simulink model "mpsimulationv5_2"  (R2025a)
settings: Solver=ode45  StartTime=0.0  StopTime=50  MaxStep=0.1  RelTol=1e-3
undefined symbols (not defined in the file): gray
libraries: dspvision x1, slpidlib x1, autolibshared x1
settings Model: Creator=shipr  LastModifiedBy=bcb

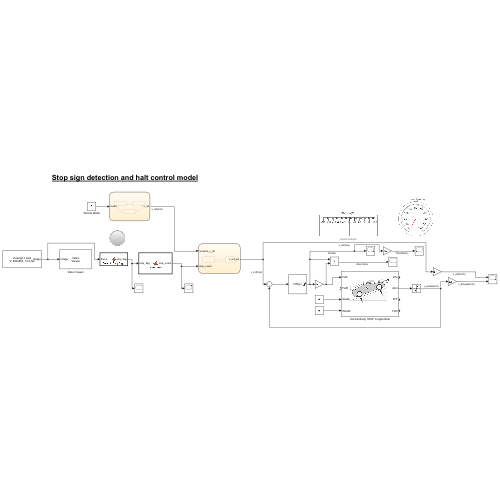
[thumbnail: Simulink's stored preview of the top-level diagram]
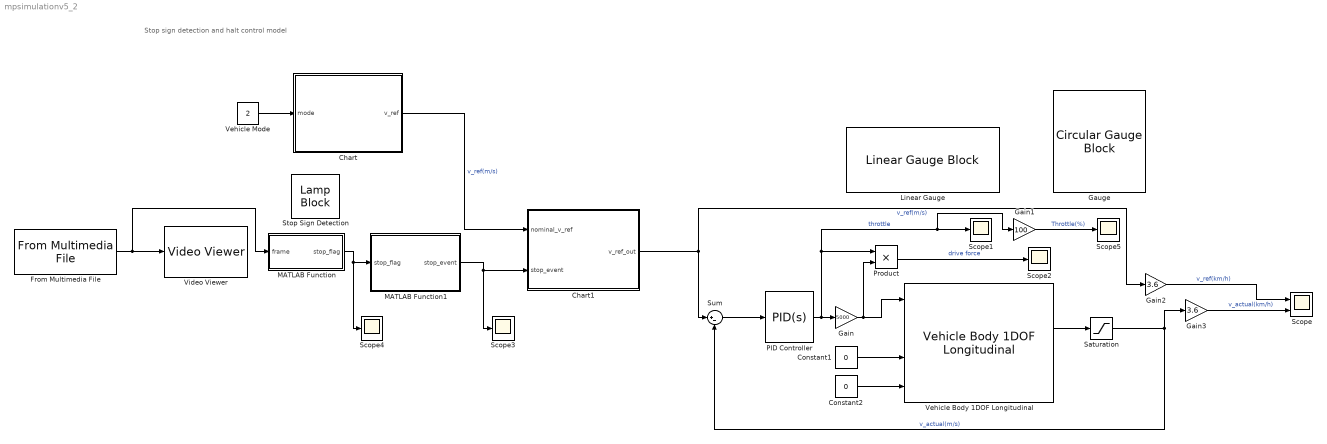
== system mpsimulationv5_2 ==
  note: Stop sign detection and halt control model
  Chart : Stateflow chart  TreatAsAtomicUnit=on
  Chart1 : Stateflow chart  TreatAsAtomicUnit=on
  Constant1 : Constant  Value=0
  Constant2 : Constant  Value=0
  From Multimedia File : dspvision/From Multimedia File  inputFilename=C:\Users\bcb\Downloads\stopsign1.mp4  readRange=[1 Inf]  loop=on  numPlays=inf  outputStreams=Video only  videoDataType=uint8  audioDataType=int16  inheritSampleTime=off  userDefinedSampleTime=0.1  noAudioOutput=off  isIntensityVideo=off  fourcc=RGB  colorVideoFormat=One multidimensional signal  outputEOF=off  dataOrg=Column-major  audioFrameSize=1024  computeAudioFrameSize=off  outSamplingMode=Sample based
      settings: LibrarySourceBlock=visionsources/From Multimedia File
  Gain : Gain  Gain=5000
  Gain1 : Gain  Gain=100
  Gain2 : Gain  Gain=3.6
  Gain3 : Gain  Gain=3.6
  Gauge : CircularGaugeBlock  FontColor=[0.0, 0.0, 0.0]
  Linear Gauge : LinearGaugeBlock  ScaleMin=-100  FontColor=[0.0, 0.0, 0.0]
  MATLAB Function : MATLAB Function  TreatAsAtomicUnit=on
  MATLAB Function1 : MATLAB Function  TreatAsAtomicUnit=on
  PID Controller : slpidlib/PID Controller  Controller=PID  Form=Parallel  TimeDomain=Continuous-time  UseExternalTs=off  SampleTime=-1  IntegratorMethod=Forward Euler  FilterMethod=Forward Euler  ControllerParametersSource=internal  P=1  I=0.1  UseKiTs=off  D=0  UseExternalDerivativeSource=off  N=100  UseFilter=on  TunerSelectOption=Transfer Function Based (PID Tuner App)  InitialConditionSource=internal  InitialConditionForIntegrator=0  InitialConditionForFilter=0  DifferentiatorICPrevScaledInput=0  ExternalReset=none  TrackingMode=off  Kt=1  LimitOutput=on  SatLimitsSource=internal  UpperSaturationLimit=1  LowerSaturationLimit=-1  LinearizeAsGain=on  AntiWindupMode=back-calculation  Kb=1  LimitIntegrator=off  UpperIntegratorSaturationLimit=inf  LowerIntegratorSaturationLimit=-inf  POutMin=[]  POutMax=[]  IOutMin=[]  IOutMax=[]  DOutMin=[]  DOutMax=[]  NOutMin=[]  NOutMax=[]  SumOutMin=[]  SumOutMax=[]  SaturationOutMin=[]  SaturationOutMax=[]  PParamMin=[]  PParamMax=[]  IParamMin=[]  IParamMax=[]  DParamMin=[]  DParamMax=[]  NParamMin=[]  NParamMax=[]  KbParamMin=[]  KbParamMax=[]  KtParamMin=[]  KtParamMax=[]  KbOutMin=[]  KbOutMax=[]  KtOutMin=[]  KtOutMax=[]  IntegratorOutMin=[]  IntegratorOutMax=[]  FilterOutMin=[]  FilterOutMax=[]  SumI1OutMin=[]  SumI1OutMax=[]  SumI2OutMin=[]  SumI2OutMax=[]  SumI3OutMin=[]  SumI3OutMax=[]  SumI4OutMin=[]  SumI4OutMax=[]  SumDOutMin=[]  SumDOutMax=[]  DifferentiatorOutMin=[]  DifferentiatorOutMax=[]  FilterDiffOutCoefMin=[]  FilterDiffOutCoefMax=[]  ReciprocalOutMin=[]  ReciprocalOutMax=[]  SumDenOutMin=[]  SumDenOutMax=[]  SumNumOutMin=[]  SumNumOutMax=[]  DivideOutMin=[]  DivideOutMax=[]  UdiffTsProdOutMin=[]  UdiffTsProdOutMax=[]  NTsProdOutMin=[]  NTsProdOutMax=[]  UintegralTsProdOutMin=[]  UintegralTsProdOutMax=[]  UngainTsProdOutMin=[]  UngainTsProdOutMax=[]  ClampingZeroOutDataTypeStr=Inherit: Inherit via back propagation  ClampingZeroOutMin=[]  ClampingZeroOutMax=[]  FilterDenConstantOutDataTypeStr=Inherit: Inherit via back propagation  FilterDenConstantOutMin=[]  FilterDenConstantOutMax=[]  PCopyOutDataTypeStr=Inherit: Inherit via back propagation  PCopyOutMin=[]  PCopyOutMax=[]  NCopyOutDataTypeStr=Inherit: Inherit via back propagation  NCopyOutMin=[]  NCopyOutMax=[]  IntegratorContinuousStateAttributes=''  IntegratorStateMustResolveToSignalObject=off  IntegratorRTWStateStorageClass=Auto  FilterContinuousStateAttributes=''  FilterStateMustResolveToSignalObject=off  FilterRTWStateStorageClass=Auto  ParallelPVariant=InternalParameters  IdealPVariant=Disabled  IVariant=InternalParameters  DVariant=InternalParameters  IntegratorVariant=Continuous  SatVariant=Enabled  AWVariant=BackCalculation  PCopyVariant=Disabled  TRVariant=Disabled  FdbkBlocksVariant=Forward  IdealPFdbkVariant=Disabled  SatFdbkVariant=Disabled  DerivativeFilterVariant=ContFilter  NVariant=InternalParameters  NCopyVariant=Disabled  FilterICVariant=InternalICsFilter  IntegratorICVariant=InternalICs  ExternalResetVariant=Disabled  TRSumVariant=Passthrough  SumFdbkVariant=Disabled  SumVariant=Sum_PID  TsampFilterVariant=InternalTs  TsampNgainVariant=Passthrough  TsampIntegralVariant=Disabled_SignalSpec  ExternalSaturationOutDataTypeStr=Inherit: Same as second input  DerivativeSourceVariant=ErrorSignal  PreIntVariant=InternalPreInt
  Product : Product
  Saturation : Saturate  UpperLimit=41.6667  LowerLimit=0
  Scope : Scope  NumInputPorts=2
      settings: Title=Velocity vs Time  ShowGrid=off  ActiveDisplayYMinimum=-327.61362751002292  ActiveDisplayYMaximum=94.622504183369685  YLabel=Velocity(km/h)
  Scope{1..5} (5 alike) : Scope
      Scope1 settings: ActiveDisplayYMinimum=-0.18455559045226133  ActiveDisplayYMaximum=1.1935694095477389
      Scope2 settings: Title=Drive Force  ActiveDisplayYMinimum=-1685.3571517954197  ActiveDisplayYMaximum=6690.2406021108291  YLabel=Drive Force  DataLoggingVariableName=ScopeData2
      Scope3 settings: ActiveDisplayYMinimum=-1.0419685990338166  ActiveDisplayYMaximum=1.0580314009661835  DataLoggingVariableName=ScopeData3
      Scope4 settings: ActiveDisplayYMinimum=-1  ActiveDisplayYMaximum=1  DataLoggingVariableName=ScopeData4
      Scope5 settings: ActiveDisplayYMinimum=-125  ActiveDisplayYMaximum=125  YLabel=Throttle (%)  DataLoggingVariableName=ScopeData5
  Stop Sign Detection : LampBlock  Tag=Stop Sign Detection  LabelPosition=Hide  DefaultColor=[192.0, 192.0, 192.0]
  Sum : Sum  Inputs=|+-
  Vehicle Body 1DOF Longitudinal : autolibshared/Vehicle Body 1DOF Longitudinal  VariantControl=SL  extFMode=off  extMMode=off  extTamb=off  wind3D=off  aMode=2  NF=2  NR=2  m=1500  a=1.4  b=1.8  h=.35  Cd=0  Cl=0  Cpm=0  Af=2.2  x_o=0  xdot_o=0  Pabs=101325  T=293  g=9.81
      settings: LibrarySourceBlock=vehdynlibeom/Vehicle Body 1DOF Longitudinal
  Vehicle Mode : Constant  Value=2
  Video Viewer : VideoViewer  colormapValue=gray(256)  FigPos=[485 762 467 342]
  wires:
  Vehicle Mode/1 -> Chart/1(mode)
  Saturation/1 -> Gain3/1, Sum/2  "v_actual(m/s)"
  Vehicle Body 1DOF Longitudinal/2 -> Saturation/1
  PID Controller/1 -> Gain1/1, Scope1/1, Product/1, Gain/1  "throttle"
  Gain/1 -> Product/2, Vehicle Body 1DOF Longitudinal/1
  Constant1/1 -> Vehicle Body 1DOF Longitudinal/3
  Constant2/1 -> Vehicle Body 1DOF Longitudinal/4
  Product/1 -> Scope2/1  "drive force"
  From Multimedia File/1 -> MATLAB Function/1(frame), Video Viewer/1
  MATLAB Function/1(stop_flag) -> Scope4/1, MATLAB Function1/1(stop_flag)
  Chart1/1(v_ref_out) -> Sum/1, Gain2/1  "v_ref(m/s)"
  Chart/1(v_ref) -> Chart1/1(nominal_v_ref)  "v_ref(m/s)"
  Sum/1 -> PID Controller/1
  MATLAB Function1/1(stop_event) -> Scope3/1, Chart1/2(stop_event)
  Gain1/1 -> Scope5/1  "Throttle(%)"
  Gain2/1 -> Scope/1  "v_ref(km/h)"
  Gain3/1 -> Scope/2  "v_actual(km/h)"

== matlab function mpsimulationv5_2/MATLAB Function1 ==
  data: stop_flag input; stop_event output
function stop_event = Debounce(stop_flag)
% Requires N consecutive detections before triggering

persistent count
if isempty(count)
    count = 0;
end

N = 2; 
if stop_flag
    count = count + 1;
else
    count = 0;
end

stop_event = (count >= N);
end

== matlab function mpsimulationv5_2/MATLAB Function ==
  data: frame input; stop_flag output
function stop_flag = Detect_StopSign(frame)
% Input:  frame - HxWx3 uint8 RGB image
% Output: stop_flag - logical true if stop sign detected

stop_flag = false;

if isempty(frame)
    return;
end

img = im2double(frame);

hsvImg = rgb2hsv(img);
H = hsvImg(:,:,1);
S = hsvImg(:,:,2);
V = hsvImg(:,:,3);

%Red color mask 
mask1 = (H < 0.08) & (S > 0.3) & (V > 0.2);
mask2 = (H > 0.88) & (S > 0.3) & (V > 0.2);
mask = mask1 | mask2;

mask = bwareaopen(mask, 200);               
mask = imclose(mask, strel('disk', 6));     

% Connected components
stats = regionprops(mask, 'Area', 'BoundingBox');

% Frame size
imgH = size(mask,1); 
imgW = size(mask,2);

for k = 1:length(stats)
    if stats(k).Area > 200  
        bb = stats(k).BoundingBox; % [x y w h]
        cx = bb(1) + bb(3)/2;
        cy = bb(2) + bb(4)/2;

        if (cx > imgW*0.15) && (cx < imgW*0.85) && (cy > imgH*0.1)
            stop_flag = true;


            return;
        end
    end
end
end

== stateflow chart mpsimulationv5_2/Chart ==
  state Eco
    during: v_ref = 15;
  state Normal
    during: v_ref = 22;
  state Sport
    during: v_ref=30;
  (default) -> Eco
  Eco -> Normal [order 1] : [mode==2]
  Normal -> Eco [order 1] : [mode==1]
  Sport -> Eco [order 1] : [mode==1]
  Eco -> Sport [order 2] : [mode==3]
  Normal -> Sport [order 2] : [mode==3]
  Sport -> Normal [order 2] : [mode==2]
  data: mode input; v_ref output

== stateflow chart mpsimulationv5_2/Chart1 ==
  state Driving
    v_ref_out = nominal_v_ref;
  state Stopping
    v_ref_out = 0;
  (default) -> Driving
  Driving -> Stopping : [stop_event==1]
  Stopping -> Driving : [after(3, sec)]
  data: v_ref_out output double; nominal_v_ref input; stop_event input
